simulink model "TorqueDesacoplado"  (R2023b)
settings: Solver=VariableStepAuto  StartTime=0.0  StopTime=10.0  RelTol=1e-3
values from neighbouring files (symbols this model uses):
  b_eq = b_m + b_l/(r^2)    (= 2.19444444444e-05)    [varLC.m]
  k_l = m * L_cm + m_l * L_l    (= 1)    [varLC.m]
  L_d = 6.6 * 10^(-3)    (= 0.0066)    [varLC.m]
  L_q = 5.8 * 10^(-3)    (= 0.0058)    [varLC.m]
  lambda_m = 0.016    [varLC.m]
  P_p = 3    [Controlador.m]    (also in varLC.m)
  r = 120/1    (= 120)    [varLC.m]
settings Model: Creator=tomas  LastModifiedBy=gonza

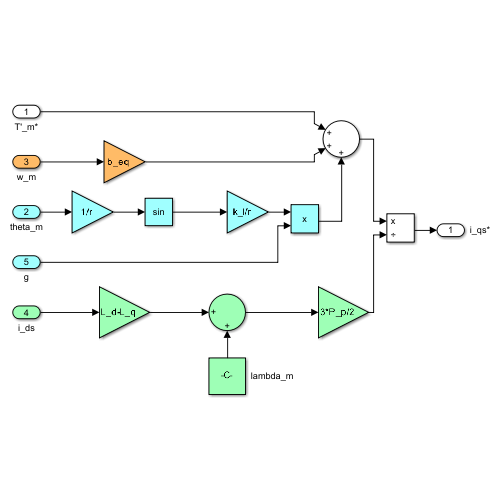
[thumbnail: Simulink's stored preview of the top-level diagram]
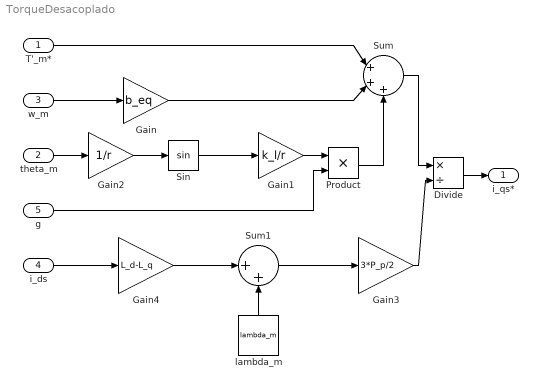
== system TorqueDesacoplado ==
  T'_m* : Inport
  theta_m : Inport  Port=2
  w_m : Inport  Port=3
  i_ds : Inport  Port=4
  g : Inport  Port=5
  Divide : Product  Inputs=*/
  Gain : Gain  Gain=b_eq
  Gain1 : Gain  Gain=k_l/r
  Gain2 : Gain  Gain=1/r
  Gain3 : Gain  Gain=3*P_p/2
  Gain4 : Gain  Gain=L_d-L_q
  Product : Product
  Sin : Trigonometry
  Sum : Sum  Inputs=|+++
  Sum1 : Sum  Inputs=|++
  lambda_m : Constant  Value=lambda_m
  i_qs* : Outport
  wires:
  Divide/1 -> i_qs*/1
  T'_m*/1 -> Sum/1
  w_m/1 -> Gain/1
  Gain/1 -> Sum/2
  Gain1/1 -> Product/1
  g/1 -> Product/2
  Product/1 -> Sum/3
  Sum/1 -> Divide/1
  Gain2/1 -> Sin/1
  theta_m/1 -> Gain2/1
  Sin/1 -> Gain1/1
  Gain3/1 -> Divide/2
  i_ds/1 -> Gain4/1
  Sum1/1 -> Gain3/1
  Gain4/1 -> Sum1/1
  lambda_m/1 -> Sum1/2
